simulink model "model1"  (R2018b)
settings: Solver=ode4  StartTime=0.0  StopTime=10.0  FixedStep=0.01  RelTol=1e-3
values from neighbouring files (symbols this model uses):
  c_c = 15000    [dane.m]
  c_w = 200000    [dane.m]
  d_c = 200    [dane.m]
  d_w = 100    [dane.m]
  m_c = 250    [dane.m]
  m_w = 30    [dane.m]
settings Model: Creator=lpa1  LastModifiedBy=Admin

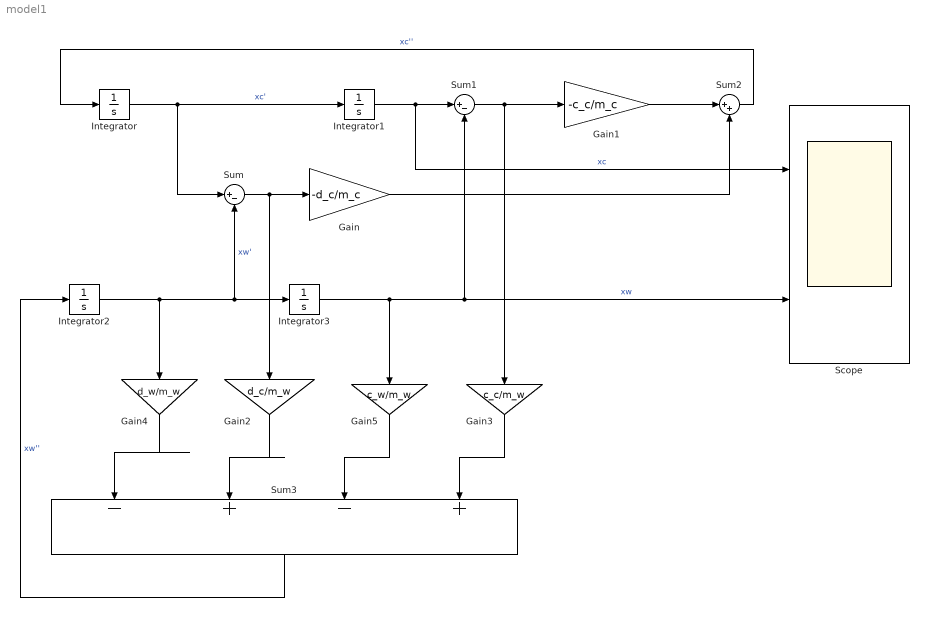
== system model1 ==
  Gain : Gain  Gain=-d_c/m_c
  Gain1 : Gain  Gain=-c_c/m_c
  Gain2 : Gain  Gain=d_c/m_w
  Gain3 : Gain  Gain=c_c/m_w
  Gain4 : Gain  Gain=d_w/m_w
  Gain5 : Gain  Gain=c_w/m_w
  Integrator : Integrator
  Integrator1 : Integrator  InitialCondition=1
  Integrator2 : Integrator
  Integrator3 : Integrator  InitialCondition=1
  Scope : Scope  NumInputPorts=2
  Sum : Sum  Inputs=|+-
  Sum1 : Sum  Inputs=|+-
  Sum2 : Sum  Inputs=|++
  Sum3 : Sum  Inputs=|-+-+
  wires:
  Integrator/1 -> Sum/1, Integrator1/1  "xc'"
  Integrator2/1 -> Integrator3/1, Sum/2, Gain4/1  "xw'"
  Sum/1 -> Gain/1, Gain2/1
  Integrator1/1 -> Scope/1, Sum1/1  "xc"
  Integrator3/1 -> Gain5/1, Scope/2, Sum1/2  "xw"
  Sum1/1 -> Gain1/1, Gain3/1
  Gain/1 -> Sum2/2
  Gain1/1 -> Sum2/1
  Sum2/1 -> Integrator/1  "xc''"
  Gain4/1 -> Sum3/1
  Gain2/1 -> Sum3/2
  Gain3/1 -> Sum3/4
  Gain5/1 -> Sum3/3
  Sum3/1 -> Integrator2/1  "xw''"
